simulink model "zynqRadioHWSWLTEMIBDetectorRFSoC2x2"  (R2022a)
settings: Solver=FixedStepDiscrete  StartTime=0.0  StopTime=2*simParams.stopTime  RelTol=1e-3
PreLoadFcn:
  | zynqRadioHWSWLTEInit;
InitFcn:
  | zynqRadioHWSWLTEInit;
undefined symbols (not defined in the file): dlDetConfig, resample, simParams, tb_dataIn, testWaveformData, testWaveformLength
libraries: dspsigops x13, simulink x5, xilinxrfsoclib x4, dspsrcs4 x2, dspmlti4 x2, hdlsllib x2, dsphdlfiltering2 x1
settings Model: DataTypeOverride=Off  SimulationMode=accelerator  Creator=The MathWorks, Inc.  LastModifiedBy=pshubh
settings SolverCC: AlgebraicLoopSolver=TrustRegion
settings DataIOCC: LimitDataPoints=on  SaveFormat=Array  SaveOutput=off  VisualizeSimOutput=off  SaveTime=off  ReturnWorkspaceOutputs=off
settings OptimizationCC: BlockReduction=off  BooleanDataType=off  ConditionallyExecuteInputs=off  DefaultParameterBehavior=Inlined  InheritOutputTypeSmallerThanSingle=on  EfficientMapNaN2IntZero=off  LifeSpan=inf
settings DebuggingCC: AlgebraicLoopMsg=error  SaveWithParameterizedLinksMsg=none  UnderspecifiedInitializationDetection=Classic  MergeDetectMultiDrivingBlocksExec=none  SignalResolutionControl=TryResolveAllWithWarning  InheritedTsInSrcMsg=none  SingleTaskRateTransMsg=error  ParameterPrecisionLossMsg=none  UnconnectedInputMsg=warning  UnconnectedOutputMsg=warning  UnconnectedLineMsg=warning  AllowSymbolicDim=off  StrictBusMsg=ErrorOnBusTreatedAsVector  SFUnexpectedBacktrackingDiag=warning  SFNoUnconditionalDefaultTransitionDiag=warning  SFExecutionAtInitializationDiag=none  SFMachineParentedDataDiag=warning  ArithmeticOperatorsInVariantConditions=warning
settings HardwareCC: ProdBitPerPointer=32  ProdBitPerSizeT=32  ProdBitPerPtrDiffT=32  ProdLargestAtomicFloat=None  ProdIntDivRoundTo=Undefined  ProdEndianess=Unspecified  ProdWordSize=32  ProdHWDeviceType=ASIC/FPGA->ASIC/FPGA  TargetBitPerPointer=64  TargetBitPerSizeT=64  TargetBitPerPtrDiffT=64  TargetLongLongMode=on  TargetIntDivRoundTo=Zero  TargetEndianess=LittleEndian  TargetWordSize=64  TargetHWDeviceType=MATLAB Host  ProdEqTarget=off
settings ModelReferenceCC: UpdateModelReferenceTargets=IfOutOfDate  PropagateSignalLabelsOutOfModel=off
settings SFSimCC: SimUseLocalCustomCode=off
settings RTWCC: RTWUseLocalCustomCode=off
settings CodeAppCC: MaxIdLength=128  StateflowObjectComments=on
settings GRTTargetCC: TargetLangStandard=C89/C90 (ANSI)  CombineOutputUpdateFcns=off  GRTInterface=on
settings ConfigComp: CovMetricSettings=dw  CovSaveCumulativeToWorkspaceVar=on  CovSaveSingleToWorkspaceVar=on  CovExternalEMLEnable=off  CovSFcnEnable=off

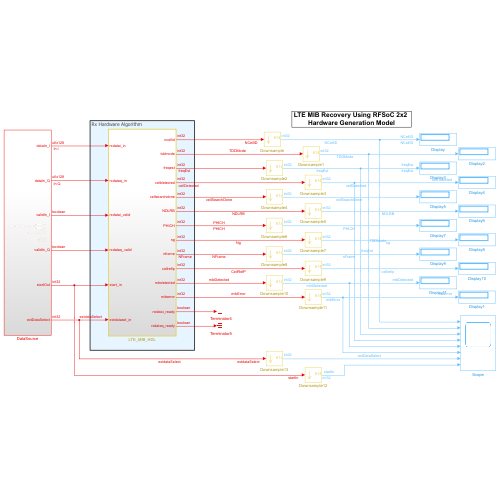
[thumbnail: Simulink's stored preview of the top-level diagram]
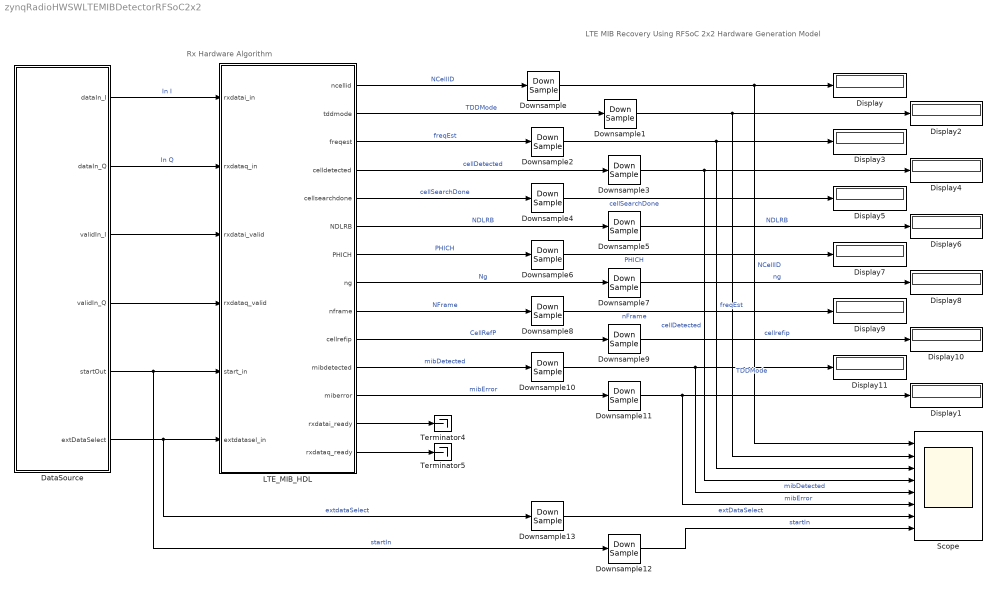
== system zynqRadioHWSWLTEMIBDetectorRFSoC2x2 ==
  note: Rx Hardware Algorithm
  note: LTE MIB Recovery Using RFSoC 2x2
      | Hardware Generation Model
  DataSource : Subsystem
  Display{,1..11} (12 alike) : Display
  Downsample{,1..13} (14 alike) : DownSample  N=61440  RateOptions=Allow multirate processing
  LTE_MIB_HDL : Subsystem  TreatAsAtomicUnit=on
  Scope : Scope  NumInputPorts=8
  Terminator4 : Terminator
  Terminator5 : Terminator
  wires:
  DataSource/4(validIn_Q) -> LTE_MIB_HDL/4(rxdataq_valid)
  DataSource/1(dataIn_I) -> LTE_MIB_HDL/1(rxdatai_in)  "In I"
  DataSource/2(dataIn_Q) -> LTE_MIB_HDL/2(rxdataq_in)  "In Q"
  DataSource/3(validIn_I) -> LTE_MIB_HDL/3(rxdatai_valid)
  LTE_MIB_HDL/5(cellsearchdone) -> Downsample4/1  "cellSearchDone"
  LTE_MIB_HDL/9(nframe) -> Downsample8/1  "NFrame"
  LTE_MIB_HDL/8(ng) -> Downsample7/1  "Ng"
  LTE_MIB_HDL/6(NDLRB) -> Downsample5/1  "NDLRB"
  LTE_MIB_HDL/10(cellrefip) -> Downsample9/1  "CellRefP"
  LTE_MIB_HDL/7(PHICH) -> Downsample6/1  "PHICH"
  LTE_MIB_HDL/3(freqest) -> Downsample2/1  "freqEst"
  DataSource/6(extDataSelect) -> Downsample13/1, LTE_MIB_HDL/6(extdatasel_in)  "extdataSelect"
  LTE_MIB_HDL/2(tddmode) -> Downsample1/1  "TDDMode"
  LTE_MIB_HDL/12(miberror) -> Downsample11/1  "mibError"
  LTE_MIB_HDL/11(mibdetected) -> Downsample10/1  "mibDetected"
  LTE_MIB_HDL/4(celldetected) -> Downsample3/1  "cellDetected"
  LTE_MIB_HDL/1(ncellid) -> Downsample/1  "NCellID"
  DataSource/5(startOut) -> Downsample12/1, LTE_MIB_HDL/5(start_in)  "startIn"
  Downsample/1 -> Display/1, Scope/1  "NCellID"
  Downsample1/1 -> Display2/1, Scope/2  "TDDMode"
  Downsample2/1 -> Display3/1, Scope/3  "freqEst"
  Downsample3/1 -> Display4/1, Scope/4  "cellDetected"
  Downsample4/1 -> Display5/1  "cellSearchDone"
  Downsample5/1 -> Display6/1  "NDLRB"
  Downsample6/1 -> Display7/1  "PHICH"
  Downsample7/1 -> Display8/1  "ng"
  Downsample8/1 -> Display9/1  "nFrame"
  Downsample9/1 -> Display10/1  "cellrefip"
  Downsample10/1 -> Display11/1, Scope/5  "mibDetected"
  Downsample11/1 -> Display1/1, Scope/6  "mibError"
  Downsample12/1 -> Scope/8  "startIn"
  Downsample13/1 -> Scope/7  "extDataSelect"
  LTE_MIB_HDL/13(rxdatai_ready) -> Terminator4/1
  LTE_MIB_HDL/14(rxdataq_ready) -> Terminator5/1

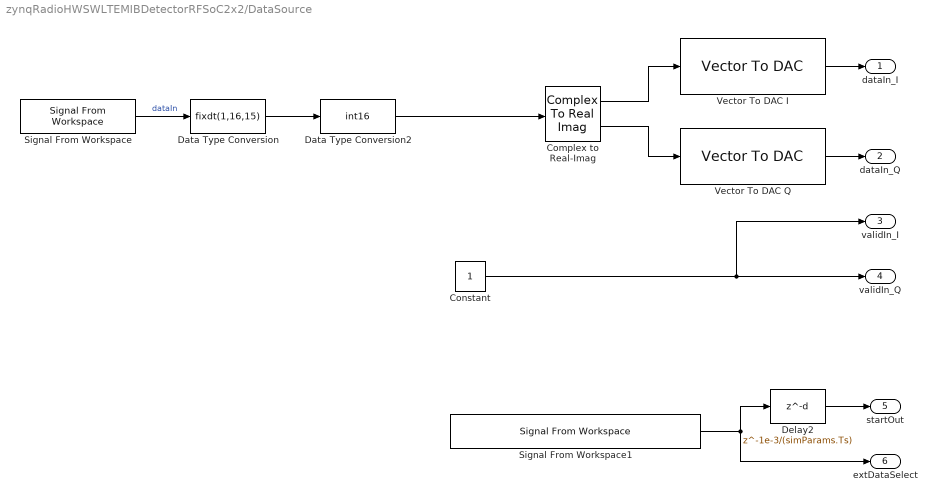
== system zynqRadioHWSWLTEMIBDetectorRFSoC2x2/DataSource ==
  Complex to Real-Imag : ComplexToRealImag
  Constant : Constant  VectorParams1D=off  OutDataTypeStr=boolean  SampleTime=simParams.Ts
  Data Type Conversion : DataTypeConversion  OutDataTypeStr=fixdt(1,16,15)  RndMeth=Floor
  Data Type Conversion2 : DataTypeConversion  OutDataTypeStr=int16  ConvertRealWorld=Stored Integer (SI)  RndMeth=Floor
  Delay2 : Delay  DelayLength=1e-3/(simParams.Ts)  InitialCondition=0
  Signal From Workspace : dspsrcs4/Signal From Workspace  X=resample(tb_dataIn,8,1)  Ts=simParams.Ts/8  nsamps=8  OutputAfterFinalValue=Cyclic repetition  ignoreOrWarnInputAndFrameLengths=on  OutputFrames=off
  Signal From Workspace1 : dspsrcs4/Signal From Workspace  X=int32([zeros(1,2457600) ones(1,3072000-2457600)])  Ts=simParams.Ts  nsamps=1  OutputAfterFinalValue=Holding final value  ignoreOrWarnInputAndFrameLengths=on  OutputFrames=off
  Vector To DAC I : xilinxrfsoclib/Vector To DAC  INPUT_WL=16  DT_INPUT=0
      settings: SourceProductBaseCode=XILINX_BLOCKSET
  Vector To DAC Q : xilinxrfsoclib/Vector To DAC  INPUT_WL=16  DT_INPUT=0
      settings: SourceProductBaseCode=XILINX_BLOCKSET
  dataIn_I : Outport
  dataIn_Q : Outport  Port=2
  validIn_I : Outport  Port=3
  validIn_Q : Outport  Port=4
  startOut : Outport  Port=5
  extDataSelect : Outport  Port=6
  wires:
  Signal From Workspace/1 -> Data Type Conversion/1  "dataIn"
  Delay2/1 -> startOut/1
  Vector To DAC I/1 -> dataIn_I/1
  Vector To DAC Q/1 -> dataIn_Q/1
  Data Type Conversion/1 -> Data Type Conversion2/1
  Complex to Real-Imag/1 -> Vector To DAC I/1
  Complex to Real-Imag/2 -> Vector To DAC Q/1
  Signal From Workspace1/1 -> Delay2/1, extDataSelect/1
  Constant/1 -> validIn_I/1, validIn_Q/1
  Data Type Conversion2/1 -> Complex to Real-Imag/1

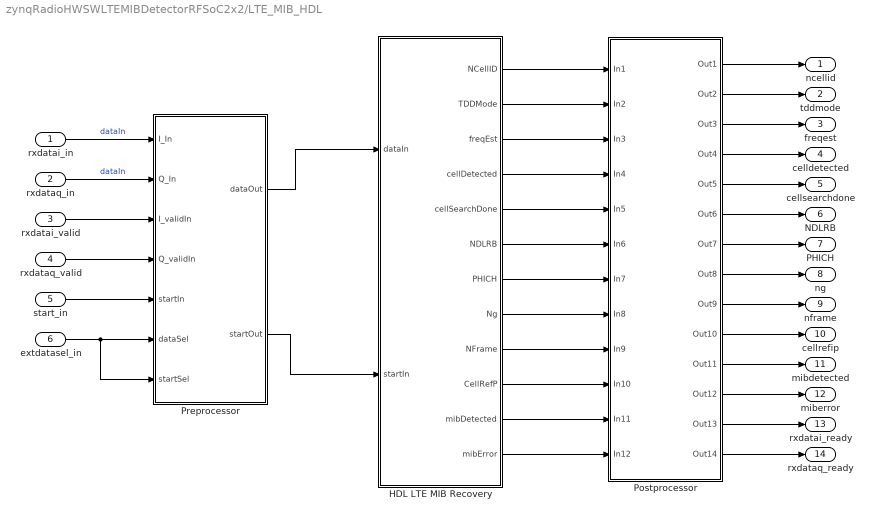
== system zynqRadioHWSWLTEMIBDetectorRFSoC2x2/LTE_MIB_HDL ==
  rxdatai_in : Inport
  rxdataq_in : Inport  Port=2
  rxdatai_valid : Inport  Port=3
  rxdataq_valid : Inport  Port=4
  start_in : Inport  Port=5
  extdatasel_in : Inport  Port=6
  HDL LTE MIB Recovery : Subsystem
  Postprocessor : Subsystem
  Preprocessor : Subsystem
  ncellid : Outport  VectorParamsAs1DForOutWhenUnconnected=off
  tddmode : Outport  Port=2  VectorParamsAs1DForOutWhenUnconnected=off
  freqest : Outport  Port=3  VectorParamsAs1DForOutWhenUnconnected=off
  celldetected : Outport  Port=4  VectorParamsAs1DForOutWhenUnconnected=off
  cellsearchdone : Outport  Port=5  VectorParamsAs1DForOutWhenUnconnected=off
  NDLRB : Outport  Port=6  VectorParamsAs1DForOutWhenUnconnected=off
  PHICH : Outport  Port=7  VectorParamsAs1DForOutWhenUnconnected=off
  ng : Outport  Port=8  VectorParamsAs1DForOutWhenUnconnected=off
  nframe : Outport  Port=9  VectorParamsAs1DForOutWhenUnconnected=off
  cellrefip : Outport  Port=10  VectorParamsAs1DForOutWhenUnconnected=off
  mibdetected : Outport  Port=11  VectorParamsAs1DForOutWhenUnconnected=off
  miberror : Outport  Port=12  VectorParamsAs1DForOutWhenUnconnected=off
  rxdatai_ready : Outport  Port=13  VectorParamsAs1DForOutWhenUnconnected=off
  rxdataq_ready : Outport  Port=14  VectorParamsAs1DForOutWhenUnconnected=off
  wires:
  Preprocessor/1(dataOut) -> HDL LTE MIB Recovery/1(dataIn)
  Preprocessor/2(startOut) -> HDL LTE MIB Recovery/2(startIn)
  rxdatai_in/1 -> Preprocessor/1(I_In)  "dataIn"
  rxdataq_in/1 -> Preprocessor/2(Q_In)  "dataIn"
  rxdatai_valid/1 -> Preprocessor/3(I_validIn)
  rxdataq_valid/1 -> Preprocessor/4(Q_validIn)
  start_in/1 -> Preprocessor/5(startIn)
  extdatasel_in/1 -> Preprocessor/7(startSel), Preprocessor/6(dataSel)
  Postprocessor/13(Out13) -> rxdatai_ready/1
  HDL LTE MIB Recovery/1(NCellID) -> Postprocessor/1(In1)
  HDL LTE MIB Recovery/2(TDDMode) -> Postprocessor/2(In2)
  HDL LTE MIB Recovery/3(freqEst) -> Postprocessor/3(In3)
  HDL LTE MIB Recovery/4(cellDetected) -> Postprocessor/4(In4)
  HDL LTE MIB Recovery/5(cellSearchDone) -> Postprocessor/5(In5)
  HDL LTE MIB Recovery/6(NDLRB) -> Postprocessor/6(In6)
  HDL LTE MIB Recovery/7(PHICH) -> Postprocessor/7(In7)
  HDL LTE MIB Recovery/8(Ng) -> Postprocessor/8(In8)
  HDL LTE MIB Recovery/9(NFrame) -> Postprocessor/9(In9)
  HDL LTE MIB Recovery/10(CellRefP) -> Postprocessor/10(In10)
  HDL LTE MIB Recovery/11(mibDetected) -> Postprocessor/11(In11)
  HDL LTE MIB Recovery/12(mibError) -> Postprocessor/12(In12)
  Postprocessor/1(Out1) -> ncellid/1
  Postprocessor/2(Out2) -> tddmode/1
  Postprocessor/3(Out3) -> freqest/1
  Postprocessor/4(Out4) -> celldetected/1
  Postprocessor/5(Out5) -> cellsearchdone/1
  Postprocessor/6(Out6) -> NDLRB/1
  Postprocessor/7(Out7) -> PHICH/1
  Postprocessor/8(Out8) -> ng/1
  Postprocessor/9(Out9) -> nframe/1
  Postprocessor/10(Out10) -> cellrefip/1
  Postprocessor/11(Out11) -> mibdetected/1
  Postprocessor/12(Out12) -> miberror/1
  Postprocessor/14(Out14) -> rxdataq_ready/1

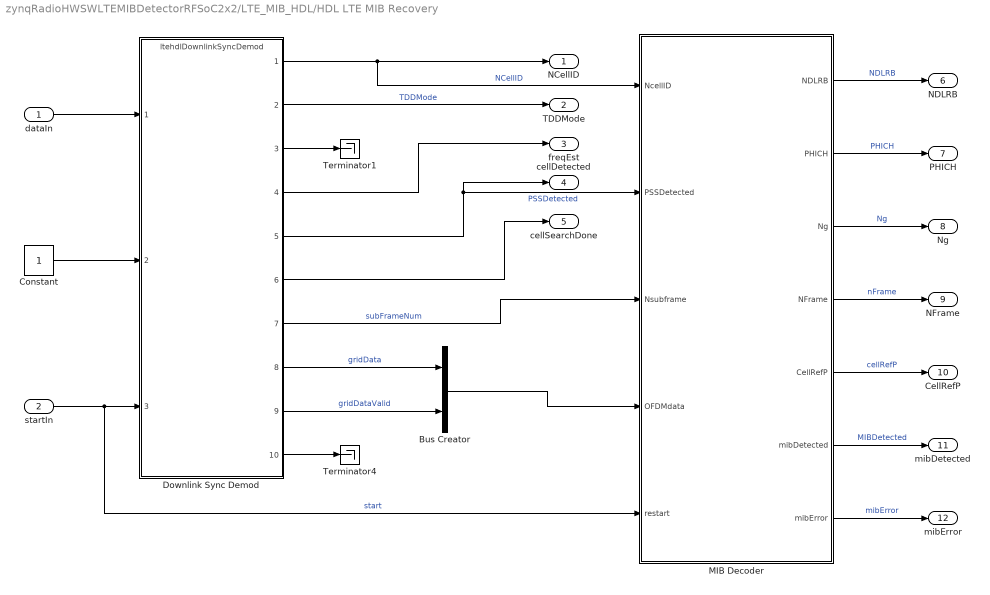
== system zynqRadioHWSWLTEMIBDetectorRFSoC2x2/LTE_MIB_HDL/HDL LTE MIB Recovery ==
  dataIn : Inport
  startIn : Inport  Port=2
  Bus Creator : BusCreator  Inputs=2  OutDataTypeStr=Bus: gridDataBus
  Constant : Constant  OutDataTypeStr=boolean  SampleTime=-1
  Downlink Sync Demod : ModelReference  ModelNameDialog=ltehdlDownlinkSyncDemod  ModelReferenceVersion=5.2
  MIB Decoder : Subsystem
  Terminator1 : Terminator
  Terminator4 : Terminator
  NCellID : Outport  PortDimensions=1  VectorParamsAs1DForOutWhenUnconnected=off
  TDDMode : Outport  Port=2  PortDimensions=1  VectorParamsAs1DForOutWhenUnconnected=off
  freqEst : Outport  Port=3  PortDimensions=1  VectorParamsAs1DForOutWhenUnconnected=off
  cellDetected : Outport  Port=4  PortDimensions=1  VectorParamsAs1DForOutWhenUnconnected=off
  cellSearchDone : Outport  Port=5  PortDimensions=1  VectorParamsAs1DForOutWhenUnconnected=off
  NDLRB : Outport  Port=6  PortDimensions=1  VectorParamsAs1DForOutWhenUnconnected=off
  PHICH : Outport  Port=7  PortDimensions=1  VectorParamsAs1DForOutWhenUnconnected=off
  Ng : Outport  Port=8  PortDimensions=1  VectorParamsAs1DForOutWhenUnconnected=off
  NFrame : Outport  Port=9  PortDimensions=1  VectorParamsAs1DForOutWhenUnconnected=off
  CellRefP : Outport  Port=10  PortDimensions=1  VectorParamsAs1DForOutWhenUnconnected=off
  mibDetected : Outport  Port=11  PortDimensions=1  VectorParamsAs1DForOutWhenUnconnected=off
  mibError : Outport  Port=12  PortDimensions=1  VectorParamsAs1DForOutWhenUnconnected=off
  wires:
  Downlink Sync Demod/7 -> MIB Decoder/3(Nsubframe)  "subFrameNum"
  MIB Decoder/6(mibDetected) -> mibDetected/1  "MIBDetected"
  Bus Creator/1 -> MIB Decoder/4(OFDMdata)
  MIB Decoder/7(mibError) -> mibError/1  "mibError"
  MIB Decoder/5(CellRefP) -> CellRefP/1  "cellRefP"
  MIB Decoder/4(NFrame) -> NFrame/1  "nFrame"
  MIB Decoder/3(Ng) -> Ng/1  "Ng"
  MIB Decoder/2(PHICH) -> PHICH/1  "PHICH"
  MIB Decoder/1(NDLRB) -> NDLRB/1  "NDLRB"
  Downlink Sync Demod/9 -> Bus Creator/2  "gridDataValid"
  Downlink Sync Demod/8 -> Bus Creator/1  "gridData"
  dataIn/1 -> Downlink Sync Demod/1
  Downlink Sync Demod/5 -> cellDetected/1, MIB Decoder/2(PSSDetected)  "PSSDetected"
  Downlink Sync Demod/1 -> NCellID/1, MIB Decoder/1(NcellID)  "NCellID"
  startIn/1 -> Downlink Sync Demod/3, MIB Decoder/5(restart)  "start"
  Downlink Sync Demod/2 -> TDDMode/1  "TDDMode"
  Downlink Sync Demod/3 -> Terminator1/1
  Downlink Sync Demod/4 -> freqEst/1
  Downlink Sync Demod/6 -> cellSearchDone/1
  Downlink Sync Demod/10 -> Terminator4/1
  Constant/1 -> Downlink Sync Demod/2

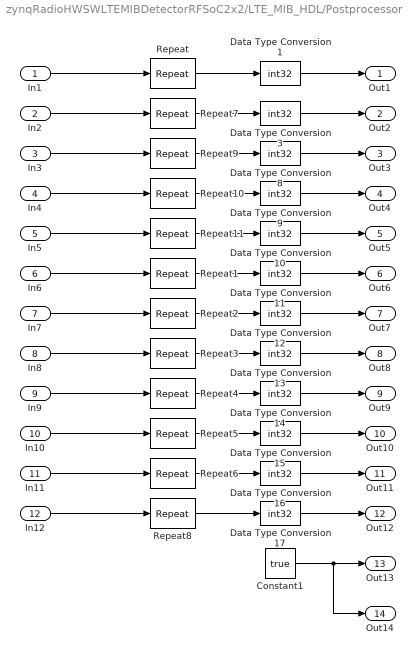
== system zynqRadioHWSWLTEMIBDetectorRFSoC2x2/LTE_MIB_HDL/Postprocessor ==
  In1 : Inport
  In2 : Inport  Port=2
  In3 : Inport  Port=3
  In4 : Inport  Port=4
  In5 : Inport  Port=5
  In6 : Inport  Port=6
  In7 : Inport  Port=7
  In8 : Inport  Port=8
  In9 : Inport  Port=9
  In10 : Inport  Port=10
  In11 : Inport  Port=11
  In12 : Inport  Port=12
  Constant1 : Constant  Value=true  VectorParams1D=off  OutDataTypeStr=boolean  SampleTime=simParams.Ts
  Data Type Conversion{1,3,8..17} (12 alike) : DataTypeConversion  OutDataTypeStr=int32  SaturateOnIntegerOverflow=off  RndMeth=Floor
  Repeat{,1..11} (12 alike) : dspsigops/Repeat  N=2  InputProcessing=Columns as channels (frame based)  RateOptions=Allow multirate processing  ic=0  mode=Unused parameter value
  Out1 : Outport
  Out2 : Outport  Port=2
  Out3 : Outport  Port=3
  Out4 : Outport  Port=4
  Out5 : Outport  Port=5
  Out6 : Outport  Port=6
  Out7 : Outport  Port=7
  Out8 : Outport  Port=8
  Out9 : Outport  Port=9
  Out10 : Outport  Port=10
  Out11 : Outport  Port=11
  Out12 : Outport  Port=12
  Out13 : Outport  Port=13
  Out14 : Outport  Port=14
  wires:
  Repeat8/1 -> Data Type Conversion17/1
  Data Type Conversion11/1 -> Out6/1
  Data Type Conversion10/1 -> Out5/1
  Repeat/1 -> Data Type Conversion1/1
  Repeat10/1 -> Data Type Conversion9/1
  Repeat9/1 -> Data Type Conversion8/1
  Repeat2/1 -> Data Type Conversion12/1
  Repeat1/1 -> Data Type Conversion11/1
  Repeat6/1 -> Data Type Conversion16/1
  Data Type Conversion1/1 -> Out1/1
  In2/1 -> Repeat7/1
  Data Type Conversion3/1 -> Out2/1
  Data Type Conversion17/1 -> Out12/1
  Repeat3/1 -> Data Type Conversion13/1
  Repeat5/1 -> Data Type Conversion15/1
  Repeat11/1 -> Data Type Conversion10/1
  Constant1/1 -> Out14/1, Out13/1
  Repeat7/1 -> Data Type Conversion3/1
  Repeat4/1 -> Data Type Conversion14/1
  In9/1 -> Repeat4/1
  In8/1 -> Repeat3/1
  In6/1 -> Repeat1/1
  In11/1 -> Repeat6/1
  Data Type Conversion9/1 -> Out4/1
  In12/1 -> Repeat8/1
  In10/1 -> Repeat5/1
  In3/1 -> Repeat9/1
  In4/1 -> Repeat10/1
  In1/1 -> Repeat/1
  Data Type Conversion14/1 -> Out9/1
  In5/1 -> Repeat11/1
  In7/1 -> Repeat2/1
  Data Type Conversion12/1 -> Out7/1
  Data Type Conversion13/1 -> Out8/1
  Data Type Conversion8/1 -> Out3/1
  Data Type Conversion15/1 -> Out10/1
  Data Type Conversion16/1 -> Out11/1

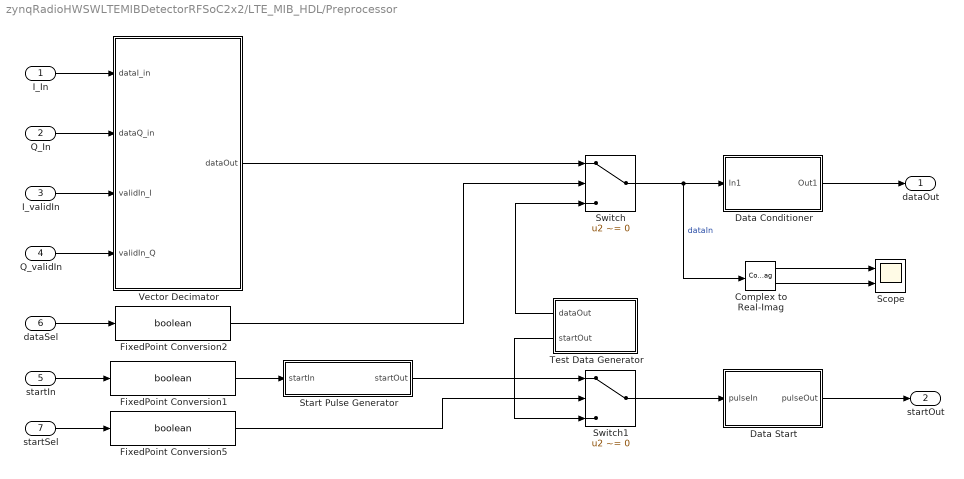
== system zynqRadioHWSWLTEMIBDetectorRFSoC2x2/LTE_MIB_HDL/Preprocessor ==
  I_In : Inport
  Q_In : Inport  Port=2
  I_validIn : Inport  Port=3
  Q_validIn : Inport  Port=4
  startIn : Inport  Port=5
  dataSel : Inport  Port=6
  startSel : Inport  Port=7
  Complex to Real-Imag : ComplexToRealImag
  Data Conditioner : Subsystem
  Data Start : Subsystem
  FixedPoint Conversion1 : DataTypeConversion  OutDataTypeStr=boolean  SaturateOnIntegerOverflow=off  RndMeth=Floor
  FixedPoint Conversion2 : DataTypeConversion  OutDataTypeStr=boolean  SaturateOnIntegerOverflow=off  RndMeth=Floor
  FixedPoint Conversion5 : DataTypeConversion  OutDataTypeStr=boolean  SaturateOnIntegerOverflow=off  RndMeth=Floor
  Scope : Scope  NumInputPorts=2
  Start Pulse Generator : Subsystem
  Switch : Switch  Criteria=u2 ~= 0  SaturateOnIntegerOverflow=off  InputSameDT=off
  Switch1 : Switch  Criteria=u2 ~= 0  SaturateOnIntegerOverflow=off  InputSameDT=off
  Test Data Generator : Subsystem  mask{framesBetweenStarts=400}
      mask prompts: framesBetweenStarts "Number of frames between start pulses"
      mask DialogControl Control2 Prompt: (min number of frames is 2)
  Vector Decimator : Subsystem
  dataOut : Outport  VectorParamsAs1DForOutWhenUnconnected=off
  startOut : Outport  Port=2  VectorParamsAs1DForOutWhenUnconnected=off
  wires:
  Test Data Generator/1(dataOut) -> Switch/3
  Test Data Generator/2(startOut) -> Switch1/3
  dataSel/1 -> FixedPoint Conversion2/1
  startIn/1 -> FixedPoint Conversion1/1
  startSel/1 -> FixedPoint Conversion5/1
  Start Pulse Generator/1(startOut) -> Switch1/1
  FixedPoint Conversion2/1 -> Switch/2
  FixedPoint Conversion1/1 -> Start Pulse Generator/1(startIn)
  FixedPoint Conversion5/1 -> Switch1/2
  Data Start/1(pulseOut) -> startOut/1
  Switch/1 -> Complex to Real-Imag/1, Data Conditioner/1(In1)  "dataIn"
  Switch1/1 -> Data Start/1(pulseIn)
  Q_validIn/1 -> Vector Decimator/4(validIn_Q)
  I_In/1 -> Vector Decimator/1(dataI_in)
  Q_In/1 -> Vector Decimator/2(dataQ_in)
  I_validIn/1 -> Vector Decimator/3(validIn_I)
  Vector Decimator/1(dataOut) -> Switch/1
  Data Conditioner/1(Out1) -> dataOut/1
  Complex to Real-Imag/1 -> Scope/1
  Complex to Real-Imag/2 -> Scope/2

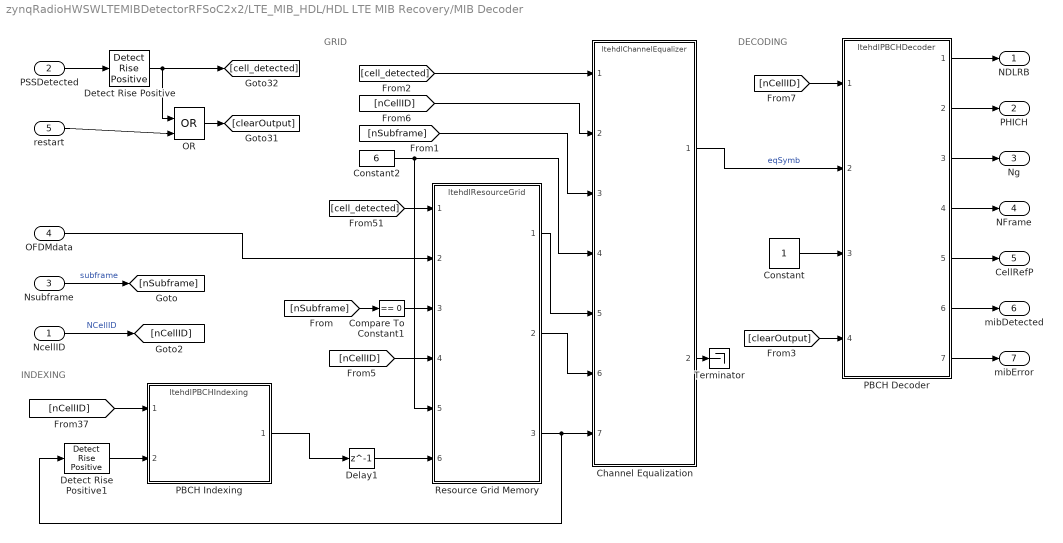
== system zynqRadioHWSWLTEMIBDetectorRFSoC2x2/LTE_MIB_HDL/HDL LTE MIB Recovery/MIB Decoder ==
  note: DECODING
  note: INDEXING
  note: GRID
  NcellID : Inport  OutDataTypeStr=fixdt(0,9,0)  PortDimensions=1
  PSSDetected : Inport  Port=2  OutDataTypeStr=boolean  PortDimensions=1
  Nsubframe : Inport  Port=3  OutDataTypeStr=fixdt(0,4,0)  PortDimensions=1
  OFDMdata : Inport  Port=4  OutDataTypeStr=Bus: gridDataBus
  restart : Inport  Port=5
  Channel Equalization : ModelReference  ModelNameDialog=ltehdlChannelEqualizer  ModelReferenceVersion=5.0
  Compare To Constant1 : simulink/Logic and Bit Operations/Compare To Constant  relop===  const=0  OutDataTypeStr=boolean
  Constant : Constant  OutDataTypeStr=boolean  SampleTime=-1
  Constant2 : Constant  Value=6  OutDataTypeStr=fixdt(0,7,0)  SampleTime=-1
  Delay1 : Delay  DelayLength=1
  Detect Rise Positive : simulink/Logic and Bit Operations/Detect Rise Positive  vinit=0  OutDataTypeStr=boolean
  Detect Rise Positive1 : simulink/Logic and Bit Operations/Detect Rise Positive  vinit=0  OutDataTypeStr=boolean
  OR : Logic  Operator=OR  IconShape=distinctive  AllPortsSameDT=off  OutDataTypeStr=boolean
  PBCH Decoder : ModelReference  ModelNameDialog=ltehdlPBCHDecoder  ModelReferenceVersion=6.0
  PBCH Indexing : ModelReference  ModelNameDialog=ltehdlPBCHIndexing  ModelReferenceVersion=6.0
  Resource Grid Memory : ModelReference  ModelNameDialog=ltehdlResourceGrid  ModelReferenceVersion=5.0
  Terminator : Terminator
  NDLRB : Outport  OutDataTypeStr=fixdt(0,7,0)  PortDimensions=1  VectorParamsAs1DForOutWhenUnconnected=off
  PHICH : Outport  Port=2  OutDataTypeStr=boolean  PortDimensions=1  VectorParamsAs1DForOutWhenUnconnected=off
  Ng : Outport  Port=3  OutDataTypeStr=fixdt(0,2,0)  PortDimensions=1  VectorParamsAs1DForOutWhenUnconnected=off
  NFrame : Outport  Port=4  OutDataTypeStr=fixdt(0,10,0)  PortDimensions=1  VectorParamsAs1DForOutWhenUnconnected=off
  CellRefP : Outport  Port=5  OutDataTypeStr=fixdt(0,3,0)  PortDimensions=1  VectorParamsAs1DForOutWhenUnconnected=off
  mibDetected : Outport  Port=6  OutDataTypeStr=boolean  PortDimensions=1  VectorParamsAs1DForOutWhenUnconnected=off
  mibError : Outport  Port=7  OutDataTypeStr=boolean  PortDimensions=1  VectorParamsAs1DForOutWhenUnconnected=off
  wires:
  PBCH Decoder/1 -> NDLRB/1
  PBCH Decoder/3 -> Ng/1
  Compare To Constant1/1 -> Resource Grid Memory/3
  PBCH Decoder/7 -> mibError/1
  Constant2/1 -> Channel Equalization/4, Resource Grid Memory/5
  PBCH Decoder/2 -> PHICH/1
  Channel Equalization/1 -> PBCH Decoder/2  "eqSymb"
  PBCH Indexing/1 -> Delay1/1
  [nCellID] -> PBCH Indexing/1
  [cell_detected] -> Resource Grid Memory/1
  PBCH Decoder/6 -> mibDetected/1
  [nCellID] -> PBCH Decoder/1
  Delay1/1 -> Resource Grid Memory/6
  Constant/1 -> PBCH Decoder/3
  Nsubframe/1 -> [nSubframe]  "subframe"
  PBCH Decoder/5 -> CellRefP/1
  PBCH Decoder/4 -> NFrame/1
  OFDMdata/1 -> Resource Grid Memory/2
  PSSDetected/1 -> Detect Rise Positive/1
  NcellID/1 -> [nCellID]  "NCellID"
  [nCellID] -> Resource Grid Memory/4
  Resource Grid Memory/3 -> Detect Rise Positive1/1, Channel Equalization/7
  Detect Rise Positive1/1 -> PBCH Indexing/2
  [nSubframe] -> Compare To Constant1/1
  [clearOutput] -> PBCH Decoder/4
  OR/1 -> [clearOutput]
  restart/1 -> OR/2
  Detect Rise Positive/1 -> [cell_detected], OR/1
  Resource Grid Memory/2 -> Channel Equalization/6
  Resource Grid Memory/1 -> Channel Equalization/5
  [cell_detected] -> Channel Equalization/1
  [nCellID] -> Channel Equalization/2
  [nSubframe] -> Channel Equalization/3
  Channel Equalization/2 -> Terminator/1

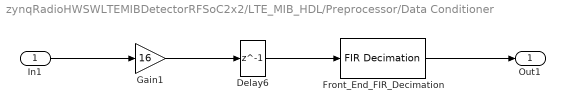
== system zynqRadioHWSWLTEMIBDetectorRFSoC2x2/LTE_MIB_HDL/Preprocessor/Data Conditioner ==
  In1 : Inport
  Delay6 : Delay  DelayLength=1  InitialCondition=0
  Front_End_FIR_Decimation : dspmlti4/FIR Decimation  FilterSource=Dialog parameters  h=dlDetConfig.frontEndFIRDecim.Numerator  D=dlDetConfig.frontEndFIRDecim.DecimationFactor  filtStruct=Direct form transposed  FilterObject=simParams.frontEndFIRDecim  framing=Enforce single-rate processing  inputOffset=0  outputBufInitCond=0  roundingMode=Floor  overflowMode=off  firstCoeffDataTypeStr=Inherit: Same word length as input  firstCoeffMin=[]  firstCoeffMax=[]  firstCoeffLastDataTypeStr=Inherit: Same word length as input  outputMode=Binary point scaling  outputWordLength=16  outputFracLength=15  outputDataTypeStr=fixdt(1,16,15)  outputMin=[]  outputMax=[]  outputLastDataTypeStr=fixdt(1,16,15)
      settings: LockScale=on
  Gain1 : Gain  Gain=16  SaturateOnIntegerOverflow=on  OutDataTypeStr=Inherit: Same as input
  Out1 : Outport
  wires:
  Gain1/1 -> Delay6/1
  Delay6/1 -> Front_End_FIR_Decimation/1
  In1/1 -> Gain1/1
  Front_End_FIR_Decimation/1 -> Out1/1

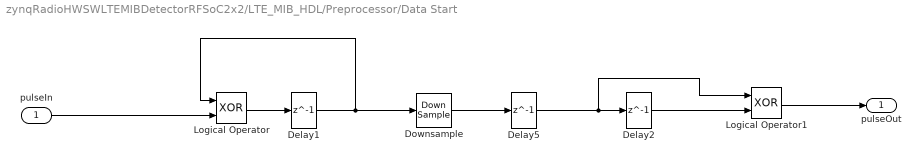
== system zynqRadioHWSWLTEMIBDetectorRFSoC2x2/LTE_MIB_HDL/Preprocessor/Data Start ==
  pulseIn : Inport
  Delay1 : Delay  DelayLength=1  InitialCondition=0
  Delay2 : Delay  DelayLength=1  InitialCondition=0
  Delay5 : Delay  DelayLength=1  InitialCondition=0
  Downsample : DownSample  RateOptions=Allow multirate processing
  Logical Operator : Logic  Operator=XOR  AllPortsSameDT=off  OutDataTypeStr=boolean
  Logical Operator1 : Logic  Operator=XOR  AllPortsSameDT=off  OutDataTypeStr=boolean
  pulseOut : Outport  VectorParamsAs1DForOutWhenUnconnected=off
  wires:
  Downsample/1 -> Delay5/1
  Delay5/1 -> Logical Operator1/1, Delay2/1
  pulseIn/1 -> Logical Operator/2
  Logical Operator/1 -> Delay1/1
  Delay1/1 -> Logical Operator/1, Downsample/1
  Logical Operator1/1 -> pulseOut/1
  Delay2/1 -> Logical Operator1/2

== system zynqRadioHWSWLTEMIBDetectorRFSoC2x2/LTE_MIB_HDL/Preprocessor/Start Pulse Generator ==
  startIn : Inport
  Delay : Delay  DelayLength=1
  Logical Operator1 : Logic  Operator=XOR  AllPortsSameDT=off  OutDataTypeStr=boolean
  Logical Operator2 : Logic  AllPortsSameDT=off  OutDataTypeStr=boolean
  startOut : Outport
  wires:
  Delay/1 -> Logical Operator1/2
  Logical Operator1/1 -> Logical Operator2/2
  startIn/1 -> Logical Operator2/1, Logical Operator1/1, Delay/1
  Logical Operator2/1 -> startOut/1

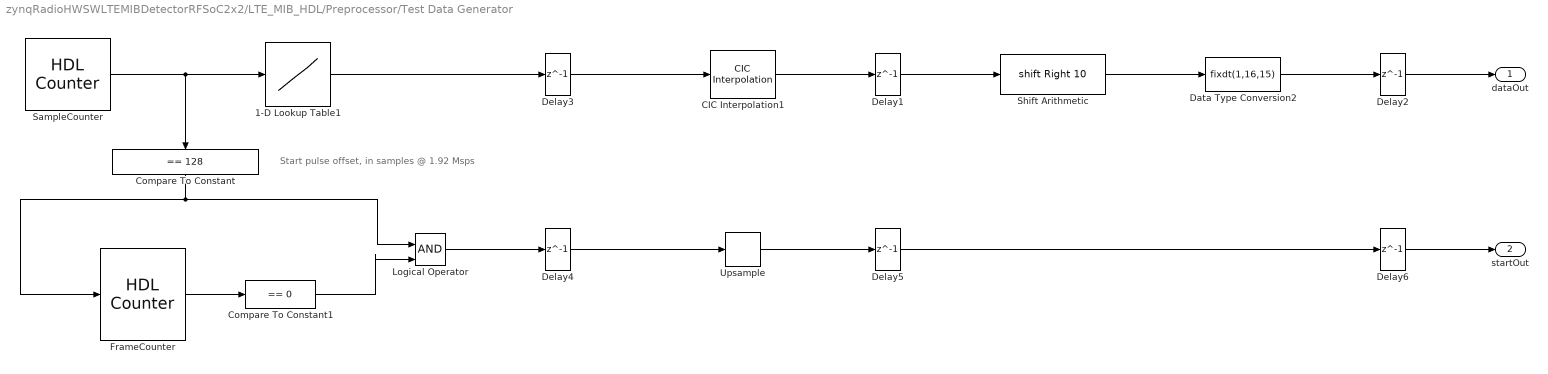
== system zynqRadioHWSWLTEMIBDetectorRFSoC2x2/LTE_MIB_HDL/Preprocessor/Test Data Generator ==
  note: Start pulse offset, in samples @ 1.92 Msps
  1-D Lookup Table1 : Lookup_n-D  NumberOfTableDimensions=1  BreakpointsSpecification=Even spacing  BreakpointsForDimension1=[-5:5]  BreakpointsForDimension1FirstPoint=0  BreakpointsForDimension2FirstPoint=10  BreakpointsForDimension2Spacing=12  IndexSearchMethod=Evenly spaced points  Table=testWaveformData  TableDataTypeStr=testWaveformData.numerictype  InterpMethod=Flat  DiagnosticForOutOfRangeInput=Error  InternalRulePriority=Speed  OutDataTypeStr=testWaveformData.numerictype  RndMeth=Simplest
  CIC Interpolation1 : dspmlti4/CIC Interpolation  filtFrom=Dialog parameters  filtobj=Hm_interp  ftype=Interpolator  R=32  M=1  N=3  filterInternals=Full precision  BPS=[16 16 16 16]  FLPS=0  outputWordLength=32  outputFracLength=0  launchFVT=off  framing=Allow multirate processing  OutputFrames=off
      settings: SourceProductBaseCode=DS
  Compare To Constant : simulink/Logic and Bit Operations/Compare To Constant  relop===  const=128  OutDataTypeStr=boolean
  Compare To Constant1 : simulink/Logic and Bit Operations/Compare To Constant  relop===  const=0  OutDataTypeStr=boolean
  Data Type Conversion2 : DataTypeConversion  OutDataTypeStr=fixdt(1,16,15)  SaturateOnIntegerOverflow=off  RndMeth=Floor
  Delay{1..6} (6 alike) : Delay  DelayLength=1  InitialCondition=0  UseCircularBuffer=on
  FrameCounter : hdlsllib/Sources/HDL Counter  CountType=Count limited  CountInit=0  CountStep=1  CountMax=framesBetweenStarts-1  CountFromType=Initial value  CountFrom=0  CountResetPort=off  CountLoadPort=off  CountEnbPort=on  CountDirPort=off  CountHitOutputPort=off  CountDataType=Unsigned  CountWordLen=nextpow2(framesBetweenStarts)  CountFracLen=0  CountSampTime=32 * simParams.Ts
  Logical Operator : Logic  IconShape=distinctive  AllPortsSameDT=off  OutDataTypeStr=boolean
  SampleCounter : hdlsllib/Sources/HDL Counter  CountType=Count limited  CountInit=0  CountStep=1  CountMax=testWaveformLength-1  CountFromType=Initial value  CountFrom=0  CountResetPort=off  CountLoadPort=off  CountEnbPort=off  CountDirPort=off  CountHitOutputPort=off  CountDataType=Unsigned  CountWordLen=nextpow2(testWaveformLength)  CountFracLen=0  CountSampTime=32 * simParams.Ts
  Shift Arithmetic : ArithShift  BitShiftNumber=10  BitShiftDirection=Right
  Upsample : dspsigops/Upsample  N=32  phase=0  RateOptions=Allow multirate processing  ic=0  mode=Unused parameter value
  dataOut : Outport  VectorParamsAs1DForOutWhenUnconnected=off
  startOut : Outport  Port=2  VectorParamsAs1DForOutWhenUnconnected=off
  wires:
  Data Type Conversion2/1 -> Delay2/1
  CIC Interpolation1/1 -> Delay1/1
  Shift Arithmetic/1 -> Data Type Conversion2/1
  SampleCounter/1 -> 1-D Lookup Table1/1, Compare To Constant/1
  1-D Lookup Table1/1 -> Delay3/1
  Delay3/1 -> CIC Interpolation1/1
  Delay1/1 -> Shift Arithmetic/1
  Delay2/1 -> dataOut/1
  Delay4/1 -> Upsample/1
  Upsample/1 -> Delay5/1
  Delay5/1 -> Delay6/1
  Compare To Constant/1 -> Logical Operator/1, FrameCounter/1
  FrameCounter/1 -> Compare To Constant1/1
  Compare To Constant1/1 -> Logical Operator/2
  Logical Operator/1 -> Delay4/1
  Delay6/1 -> startOut/1

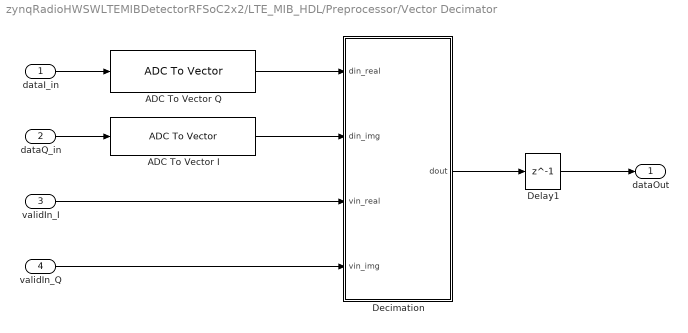
== system zynqRadioHWSWLTEMIBDetectorRFSoC2x2/LTE_MIB_HDL/Preprocessor/Vector Decimator ==
  dataI_in : Inport
  dataQ_in : Inport  Port=2
  validIn_I : Inport  Port=3  SampleTime=1/(61.44e6)
  validIn_Q : Inport  Port=4  SampleTime=1/(61.44e6)
  ADC To Vector I : xilinxrfsoclib/ADC To Vector  samplesPerClock=8  DT=fixdt(1,16,15)  INPUT_DT=0
      settings: SourceProductBaseCode=XILINX_BLOCKSET
  ADC To Vector Q : xilinxrfsoclib/ADC To Vector  samplesPerClock=8  DT=fixdt(1,16,15)  INPUT_DT=0
      settings: SourceProductBaseCode=XILINX_BLOCKSET
  Decimation : Subsystem
  Delay1 : Delay  DelayLength=1
  dataOut : Outport
  wires:
  validIn_Q/1 -> Decimation/4(vin_img)
  ADC To Vector Q/1 -> Decimation/1(din_real)
  ADC To Vector I/1 -> Decimation/2(din_img)
  validIn_I/1 -> Decimation/3(vin_real)
  Decimation/1(dout) -> Delay1/1
  Delay1/1 -> dataOut/1
  dataI_in/1 -> ADC To Vector Q/1
  dataQ_in/1 -> ADC To Vector I/1

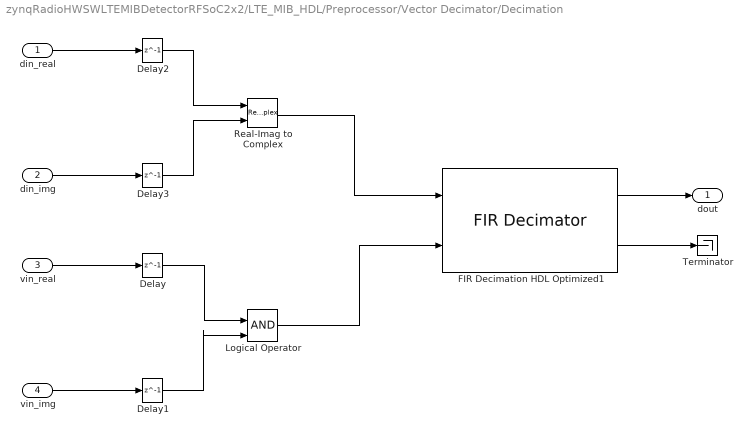
== system zynqRadioHWSWLTEMIBDetectorRFSoC2x2/LTE_MIB_HDL/Preprocessor/Vector Decimator/Decimation ==
  din_real : Inport
  din_img : Inport  Port=2
  vin_real : Inport  Port=3
  vin_img : Inport  Port=4
  Delay{,1..3} (4 alike) : Delay  DelayLength=1  InitialCondition=0
  FIR Decimation HDL Optimized1 : dsphdlfiltering2/FIR Decimator  Numerator=fir1(35,0.4)  FilterStructure=Direct form systolic  DecimationFactor=8  NumCycles=1  SimulateUsing=Code generation  roundingMode=Floor  overflowMode=off  CoefficientsDataTypeStr=Inherit: Same word length as input  OutputDataTypeStr=fixdt(1,16,15)  ResetInputPort=off  HDLGlobalReset=off
      settings: SourceProductBaseCode=HS
  Logical Operator : Logic  IconShape=distinctive  AllPortsSameDT=off  OutDataTypeStr=boolean
  Real-Imag to Complex : RealImagToComplex
  Terminator : Terminator
  dout : Outport  VectorParamsAs1DForOutWhenUnconnected=off
  wires:
  FIR Decimation HDL Optimized1/1 -> dout/1
  vin_real/1 -> Delay/1
  vin_img/1 -> Delay1/1
  din_real/1 -> Delay2/1
  din_img/1 -> Delay3/1
  Real-Imag to Complex/1 -> FIR Decimation HDL Optimized1/1
  Logical Operator/1 -> FIR Decimation HDL Optimized1/2
  Delay/1 -> Logical Operator/1
  Delay1/1 -> Logical Operator/2
  Delay2/1 -> Real-Imag to Complex/1
  Delay3/1 -> Real-Imag to Complex/2
  FIR Decimation HDL Optimized1/2 -> Terminator/1
